simulink model "testexp1_cs"  (Simulink 8.8)
settings: Solver=ode5  StartTime=0.0  StopTime=inf  FixedStep=1/20  RelTol=1e-3
model workspace (MAT data in the model file):
  mbox_table.block_array(1).src = 'built-in/Subsystem'
  mbox_table.block_array(1).dest = 'testexp1_cs/Ford_FocusWagon_1'
  mbox_table.block_array(1).mode = 0
  mbox_table.block_array(2).src = 'simulink/Sinks/Out1'
  mbox_table.block_array(2).dest = 'testexp1_cs/Ford_FocusWagon_1/STATE_Ford_FocusWagon_1'
  mbox_table.block_array(2).mode = 0
  mbox_table.block_array(3).src = 'PreScanSimulinkLibrary/State'
  mbox_table.block_array(3).dest = 'testexp1_cs/STATE_Ford_FocusWagon_1'
  mbox_table.block_array(3).mode = 0
  mbox_table.block_array(4).src = 'PreScanSimulinkLibrary/SELF'
  mbox_table.block_array(4).dest = 'testexp1_cs/SELF_Ford_FocusWagon_1'
  mbox_table.block_array(4).mode = 0
  mbox_table.block_array(5).src = 'simulink/Sources/In1'
  mbox_table.block_array(5).dest = 'testexp1_cs/Ford_FocusWagon_1/SELF_Ford_FocusWagon_1'
  mbox_table.block_array(5).mode = 0
  mbox_table.block_array(6).src = 'PreScanSimulinkLibrary/DemuxSELF'
  mbox_table.block_array(6).dest = 'testexp1_cs/Ford_FocusWagon_1/SELF_Demux'
  mbox_table.block_array(6).mode = 0
  mbox_table.block_array(7).src = 'PreScanSimulinkLibrary/UserSpecified_Subsys'
  mbox_table.block_array(7).dest = 'testexp1_cs/Ford_FocusWagon_1/Dynamics_UserSpecified'
  mbox_table.block_array(7).mode = 0
  mbox_table.block_array(8).src = 'PreScanSimulinkLibrary/MuxState'
  mbox_table.block_array(8).dest = 'testexp1_cs/Ford_FocusWagon_1/Dynamics_UserSpecified/MuxState'
  mbox_table.block_array(8).mode = 0
  mbox_table.block_array(9).src = 'simulink/Sinks/Out1'
  mbox_table.block_array(9).dest = 'testexp1_cs/Ford_FocusWagon_1/Dynamics_UserSpecified/State'
  mbox_table.block_array(9).mode = 0
  mbox_table.block_array(10).src = 'built-in/Note'
  mbox_table.block_array(10).dest = 'testexp1_cs/Ford_FocusWagon_1/Dynamics_UserSpecified/For state mode ''Dynamic'' positions
    | are not taken into account, as they
    | are computed by integrating velocity.
    | Click annotation for Help.'
  mbox_table.block_array(10).mode = 0
  mbox_table.block_array(11).src = 'SimCoreLibrary/SimCoreConfiguration'
  mbox_table.block_array(11).dest = 'testexp1_cs/SimCoreConfiguration'
  mbox_table.block_array(11).mode = 0
  mbox_table.block_array(12).src = 'SimCoreLibrary/Actuators'
  mbox_table.block_array(12).dest = 'testexp1_cs/Actuators'
  mbox_table.block_array(12).mode = 0
  mbox_table.block_array(13).src = 'SimCoreLibrary/SetActuators'
  mbox_table.block_array(13).dest = 'testexp1_cs/SetActuators'
  mbox_table.block_array(13).mode = 0
  mbox_table.block_array(14).src = 'SimCoreLibrary/GetSensors'
  mbox_table.block_array(14).dest = 'testexp1_cs/GetSensors'
  mbox_table.block_array(14).mode = 0
  mbox_table.block_array(15).src = 'SimCoreLibrary/SimCoreInfo'
  mbox_table.block_array(15).dest = 'testexp1_cs/SimCoreInfo'
  mbox_table.block_array(15).mode = 0
  mbox_table.block_array(16).src = 'PreScanSimulinkLibrary/Regenerate'
  mbox_table.block_array(16).dest = 'testexp1_cs/Regenerate'
  mbox_table.block_array(16).mode = 0
  mbox_table.block_array(17).src = 'PreScanSimulinkLibrary/Record for Replay  '
  mbox_table.block_array(17).dest = 'testexp1_cs/Record for Replay  '
  mbox_table.block_array(17).mode = 0
  mbox_table.block_array(18).src = 'PreScanSimulinkLibrary/Open Useful Blocks'
  mbox_table.block_array(18).dest = 'testexp1_cs/Open Useful Blocks'
  mbox_table.block_array(18).mode = 0
  mbox_table.block_array(19).src = 'PreScanSimulinkLibrary/PreScan Options   '
  mbox_table.block_array(19).dest = 'testexp1_cs/PreScan Options   '
  mbox_table.block_array(19).mode = 0
  mbox_table.block_array(20).src = 'built-in/Note'
  mbox_table.block_array(20).dest = 'testexp1_cs/Version:                  '
  mbox_table.block_array(20).mode = 0
  mbox_table.block_array(21).src = 'built-in/Note'
  mbox_table.block_array(21).dest = 'testexp1_cs/7.5.1'
  mbox_table.block_array(21).mode = 0
  mbox_table.block_array(22).src = 'built-in/Note'
  mbox_table.block_array(22).dest = 'testexp1_cs/Author(s):                '
  mbox_table.block_array(22).mode = 0
  mbox_table.block_array(23).src = 'built-in/Note'
  mbox_table.block_array(23).dest = 'testexp1_cs/N.A.'
  mbox_table.block_array(23).mode = 0
  mbox_table.block_array(24).src = 'built-in/Note'
  mbox_table.block_array(24).dest = 'testexp1_cs/Descriptive text:      '
  mbox_table.block_array(24).mode = 0
  mbox_table.block_array(25).src = 'built-in/Note'
  mbox_table.block_array(25).dest = 'testexp1_cs/N.A.'
  mbox_table.block_array(25).mode = 0
  mbox_table.block_array(26).src = 'built-in/Note'
  mbox_table.block_array(26).dest = 'testexp1_cs/ID
    | 
    | 2'
  mbox_table.block_array(26).mode = 0
  mbox_table.block_array(27).src = 'built-in/Note'
  mbox_table.block_array(27).dest = 'testexp1_cs/OBU-Beacon ID
    | 
    | '
  mbox_table.block_array(27).mode = 0
  mbox_table.block_array(28).src = 'built-in/Note'
  mbox_table.block_array(28).dest = 'testexp1_cs/TypeID
    | 
    | 1'
  mbox_table.block_array(28).mode = 0
  mbox_table.block_array(29).src = 'built-in/Note'
  mbox_table.block_array(29).dest = 'testexp1_cs/TypeTag
    | 
    | Car'
  mbox_table.block_array(29).mode = 0
  mbox_table.block_array(30).src = 'built-in/Note'
  mbox_table.block_array(30).dest = 'testexp1_cs/SD
    | 
    | Y'
  mbox_table.block_array(30).mode = 0
  mbox_table.block_array(31).src = 'built-in/Note'
  mbox_table.block_array(31).dest = 'testexp1_cs/CD
    | 
    | N'
  mbox_table.block_array(31).mode = 0
  mbox_table.block_array(32).src = 'built-in/Note'
  mbox_table.block_array(32).dest = 'testexp1_cs/Name
    | 
    | Ford_FocusWagon_1'
  mbox_table.block_array(32).mode = 0
  mbox_table.block_array(33).src = 'built-in/Note'
  mbox_table.block_array(33).dest = 'testexp1_cs/Num ID       OBU-Beacon ID     Type ID      Type Tag             SD        CD             Name                          '
  mbox_table.block_array(33).mode = 0
  mbox_table.block_array(34).src = 'built-in/Ground'
  mbox_table.block_array(34).dest = 'testexp1_cs/Ford_FocusWagon_1/Ground_1'
  mbox_table.block_array(34).mode = 1
  mbox_table.block_array(35).src = 'built-in/Terminator'
  mbox_table.block_array(35).dest = 'testexp1_cs/Ford_FocusWagon_1/Terminator_1'
  mbox_table.block_array(35).mode = 1
  mbox_table.block_array(36).src = 'built-in/Ground'
  mbox_table.block_array(36).dest = 'testexp1_cs/Ford_FocusWagon_1/Dynamics_UserSpecified/Ground_1'
  mbox_table.block_array(36).mode = 1
  mbox_table.block_array(37).src = 'built-in/Ground'
  mbox_table.block_array(37).dest = 'testexp1_cs/Ford_FocusWagon_1/Dynamics_UserSpecified/Ground_2'
  mbox_table.block_array(37).mode = 1
  mbox_table.block_array(38).src = 'built-in/Ground'
  mbox_table.block_array(38).dest = 'testexp1_cs/Ford_FocusWagon_1/Dynamics_UserSpecified/Ground_3'
  mbox_table.block_array(38).mode = 1
  mbox_table.block_array(39).src = 'built-in/Ground'
  mbox_table.block_array(39).dest = 'testexp1_cs/Ford_FocusWagon_1/Dynamics_UserSpecified/Ground_4'
  mbox_table.block_array(39).mode = 1
  mbox_table.block_array(40).src = 'built-in/Ground'
  mbox_table.block_array(40).dest = 'testexp1_cs/Ford_FocusWagon_1/Dynamics_UserSpecified/Ground_5'
  mbox_table.block_array(40).mode = 1
  mbox_table.block_array(41).src = 'built-in/Ground'
  mbox_table.block_array(41).dest = 'testexp1_cs/Ford_FocusWagon_1/Dynamics_UserSpecified/Ground_6'
  mbox_table.block_array(41).mode = 1
  mbox_table.block_array(42).src = 'built-in/Ground'
  mbox_table.block_array(42).dest = 'testexp1_cs/Ford_FocusWagon_1/Dynamics_UserSpecified/Ground_7'
  mbox_table.block_array(42).mode = 1
  mbox_table.block_array(43).src = 'built-in/Ground'
  mbox_table.block_array(43).dest = 'testexp1_cs/Ford_FocusWagon_1/Dynamics_UserSpecified/Ground_8'
  mbox_table.block_array(43).mode = 1
  mbox_table.block_array(44).src = 'built-in/Ground'
  mbox_table.block_array(44).dest = 'testexp1_cs/Ford_FocusWagon_1/Dynamics_UserSpecified/Ground_9'
  mbox_table.block_array(44).mode = 1
  mbox_table.block_array(45).src = 'built-in/Terminator'
  mbox_table.block_array(45).dest = 'testexp1_cs/Ford_FocusWagon_1/Dynamics_UserSpecified/Terminator_1'
  mbox_table.block_array(45).mode = 1
  mbox_table.block_array(46).src = 'built-in/Terminator'
  mbox_table.block_array(46).dest = 'testexp1_cs/Ford_FocusWagon_1/Terminator_2'
  mbox_table.block_array(46).mode = 1
  mbox_table.block_array(47).src = 'built-in/Terminator'
  mbox_table.block_array(47).dest = 'testexp1_cs/Ford_FocusWagon_1/Terminator_3'
  mbox_table.block_array(47).mode = 1
  mbox_table.block_array(48).src = 'built-in/Terminator'
  mbox_table.block_array(48).dest = 'testexp1_cs/Ford_FocusWagon_1/Terminator_4'
  mbox_table.block_array(48).mode = 1
  mbox_table.block_array(49).src = 'built-in/Terminator'
  mbox_table.block_array(49).dest = 'testexp1_cs/Ford_FocusWagon_1/Terminator_5'
  mbox_table.block_array(49).mode = 1
  mbox_table.block_array(50).src = 'built-in/Terminator'
  mbox_table.block_array(50).dest = 'testexp1_cs/Ford_FocusWagon_1/Terminator_6'
  mbox_table.block_array(50).mode = 1
  mbox_table.block_array(51).src = 'built-in/Terminator'
  mbox_table.block_array(51).dest = 'testexp1_cs/Ford_FocusWagon_1/Terminator_7'
  mbox_table.block_array(51).mode = 1
  mbox_table.block_array(52).src = 'built-in/Terminator'
  mbox_table.block_array(52).dest = 'testexp1_cs/Ford_FocusWagon_1/Terminator_8'
  mbox_table.block_array(52).mode = 1
  mbox_table.block_array(53).src = 'built-in/Terminator'
  mbox_table.block_array(53).dest = 'testexp1_cs/Ford_FocusWagon_1/Terminator_9'
  mbox_table.block_array(53).mode = 1
  mbox_table.block_array(54).src = 'built-in/Terminator'
  mbox_table.block_array(54).dest = 'testexp1_cs/Ford_FocusWagon_1/Terminator_10'
  mbox_table.block_array(54).mode = 1
  mbox_table.block_array(55).src = 'built-in/Terminator'
  mbox_table.block_array(55).dest = 'testexp1_cs/Ford_FocusWagon_1/Terminator_11'
  mbox_table.block_array(55).mode = 1
  mbox_table.block_array(56).src = 'built-in/Terminator'
  mbox_table.block_array(56).dest = 'testexp1_cs/Ford_FocusWagon_1/Terminator_12'
  mbox_table.block_array(56).mode = 1
  mbox_table.block_array(57).src = 'built-in/Terminator'
  mbox_table.block_array(57).dest = 'testexp1_cs/Ford_FocusWagon_1/Terminator_13'
  mbox_table.block_array(57).mode = 1
  mbox_table.block_index : java.util.Hashtable (value not decoded)
  mbox_table.line_array(1).sys = 'testexp1_cs'
  mbox_table.line_array(1).line_id = 'L1'
  mbox_table.line_array(1).iport = 'STATE_Ford_FocusWagon_1/1'
  mbox_table.line_array(1).oport = 'Ford_FocusWagon_1/1'
  mbox_table.line_array(1).mode = 0
  mbox_table.line_array(2).sys = 'testexp1_cs'
  mbox_table.line_array(2).line_id = 'L2'
  mbox_table.line_array(2).iport = 'Ford_FocusWagon_1/1'
  mbox_table.line_array(2).oport = 'SELF_Ford_FocusWagon_1/1'
  mbox_table.line_array(2).mode = 0
  mbox_table.line_array(3).sys = 'testexp1_cs/Ford_FocusWagon_1'
  mbox_table.line_array(3).line_id = 'L3'
  mbox_table.line_array(3).iport = 'SELF_Demux/1'
  mbox_table.line_array(3).oport = 'SELF_Ford_FocusWagon_1/1'
  mbox_table.line_array(3).mode = 0
  mbox_table.line_array(4).sys = 'testexp1_cs/Ford_FocusWagon_1/Dynamics_UserSpecified'
  mbox_table.line_array(4).line_id = 'L4'
  mbox_table.line_array(4).iport = 'State/1'
  mbox_table.line_array(4).oport = 'MuxState/1'
  mbox_table.line_array(4).mode = 0
  mbox_table.line_array(5).sys = 'testexp1_cs/Ford_FocusWagon_1'
  mbox_table.line_array(5).line_id = 'L5'
  mbox_table.line_array(5).iport = 'STATE_Ford_FocusWagon_1/1'
  mbox_table.line_array(5).oport = 'Dynamics_UserSpecified/1'
  mbox_table.line_array(5).mode = 0
  mbox_table.line_array(6).sys = 'testexp1_cs/Ford_FocusWagon_1'
  mbox_table.line_array(6).line_id = 'l1'
  mbox_table.line_array(6).iport = 'Dynamics_UserSpecified/1'
  mbox_table.line_array(6).oport = 'Ground_1/1'
  mbox_table.line_array(6).mode = 1
  mbox_table.line_array(7).sys = 'testexp1_cs/Ford_FocusWagon_1'
  mbox_table.line_array(7).line_id = 'l2'
  mbox_table.line_array(7).iport = 'Terminator_1/1'
  mbox_table.line_array(7).oport = 'Dynamics_UserSpecified/2'
  mbox_table.line_array(7).mode = 1
  mbox_table.line_array(8).sys = 'testexp1_cs/Ford_FocusWagon_1/Dynamics_UserSpecified'
  mbox_table.line_array(8).line_id = 'l3'
  mbox_table.line_array(8).iport = 'MuxState/1'
  mbox_table.line_array(8).oport = 'Ground_1/1'
  mbox_table.line_array(8).mode = 1
  mbox_table.line_array(9).sys = 'testexp1_cs/Ford_FocusWagon_1/Dynamics_UserSpecified'
  mbox_table.line_array(9).line_id = 'l4'
  mbox_table.line_array(9).iport = 'MuxState/2'
  mbox_table.line_array(9).oport = 'Ground_2/1'
  mbox_table.line_array(9).mode = 1
  mbox_table.line_array(10).sys = 'testexp1_cs/Ford_FocusWagon_1/Dynamics_UserSpecified'
  mbox_table.line_array(10).line_id = 'l5'
  mbox_table.line_array(10).iport = 'MuxState/3'
  mbox_table.line_array(10).oport = 'Ground_3/1'
  mbox_table.line_array(10).mode = 1
  mbox_table.line_array(11).sys = 'testexp1_cs/Ford_FocusWagon_1/Dynamics_UserSpecified'
  mbox_table.line_array(11).line_id = 'l6'
  mbox_table.line_array(11).iport = 'MuxState/4'
  mbox_table.line_array(11).oport = 'Ground_4/1'
  mbox_table.line_array(11).mode = 1
  mbox_table.line_array(12).sys = 'testexp1_cs/Ford_FocusWagon_1/Dynamics_UserSpecified'
  mbox_table.line_array(12).line_id = 'l7'
  mbox_table.line_array(12).iport = 'MuxState/5'
  mbox_table.line_array(12).oport = 'Ground_5/1'
  mbox_table.line_array(12).mode = 1
  mbox_table.line_array(13).sys = 'testexp1_cs/Ford_FocusWagon_1/Dynamics_UserSpecified'
  mbox_table.line_array(13).line_id = 'l8'
  mbox_table.line_array(13).iport = 'MuxState/6'
  mbox_table.line_array(13).oport = 'Ground_6/1'
  mbox_table.line_array(13).mode = 1
  mbox_table.line_array(14).sys = 'testexp1_cs/Ford_FocusWagon_1/Dynamics_UserSpecified'
  mbox_table.line_array(14).line_id = 'l9'
  mbox_table.line_array(14).iport = 'MuxState/7'
  mbox_table.line_array(14).oport = 'Ground_7/1'
  mbox_table.line_array(14).mode = 1
  mbox_table.line_array(15).sys = 'testexp1_cs/Ford_FocusWagon_1/Dynamics_UserSpecified'
  mbox_table.line_array(15).line_id = 'l10'
  mbox_table.line_array(15).iport = 'MuxState/8'
  mbox_table.line_array(15).oport = 'Ground_8/1'
  mbox_table.line_array(15).mode = 1
  mbox_table.line_array(16).sys = 'testexp1_cs/Ford_FocusWagon_1/Dynamics_UserSpecified'
  mbox_table.line_array(16).line_id = 'l11'
  mbox_table.line_array(16).iport = 'MuxState/9'
  mbox_table.line_array(16).oport = 'Ground_9/1'
  mbox_table.line_array(16).mode = 1
  mbox_table.line_array(17).sys = 'testexp1_cs/Ford_FocusWagon_1/Dynamics_UserSpecified'
  mbox_table.line_array(17).line_id = 'l12'
  mbox_table.line_array(17).iport = 'Terminator_1/1'
  mbox_table.line_array(17).oport = 'Sine Wave/1'
  mbox_table.line_array(17).mode = 1
  mbox_table.line_array(18).sys = 'testexp1_cs/Ford_FocusWagon_1'
  mbox_table.line_array(18).line_id = 'l13'
  mbox_table.line_array(18).iport = 'Terminator_2/1'
  mbox_table.line_array(18).oport = 'SELF_Demux/1'
  mbox_table.line_array(18).mode = 1
  mbox_table.line_array(19).sys = 'testexp1_cs/Ford_FocusWagon_1'
  mbox_table.line_array(19).line_id = 'l14'
  mbox_table.line_array(19).iport = 'Terminator_3/1'
  mbox_table.line_array(19).oport = 'SELF_Demux/2'
  mbox_table.line_array(19).mode = 1
  mbox_table.line_array(20).sys = 'testexp1_cs/Ford_FocusWagon_1'
  mbox_table.line_array(20).line_id = 'l15'
  mbox_table.line_array(20).iport = 'Terminator_4/1'
  mbox_table.line_array(20).oport = 'SELF_Demux/3'
  mbox_table.line_array(20).mode = 1
  mbox_table.line_array(21).sys = 'testexp1_cs/Ford_FocusWagon_1'
  mbox_table.line_array(21).line_id = 'l16'
  mbox_table.line_array(21).iport = 'Terminator_5/1'
  mbox_table.line_array(21).oport = 'SELF_Demux/4'
  mbox_table.line_array(21).mode = 1
  mbox_table.line_array(22).sys = 'testexp1_cs/Ford_FocusWagon_1'
  mbox_table.line_array(22).line_id = 'l17'
  mbox_table.line_array(22).iport = 'Terminator_6/1'
  mbox_table.line_array(22).oport = 'SELF_Demux/5'
  mbox_table.line_array(22).mode = 1
  mbox_table.line_array(23).sys = 'testexp1_cs/Ford_FocusWagon_1'
  mbox_table.line_array(23).line_id = 'l18'
  mbox_table.line_array(23).iport = 'Terminator_7/1'
  mbox_table.line_array(23).oport = 'SELF_Demux/6'
  mbox_table.line_array(23).mode = 1
  mbox_table.line_array(24).sys = 'testexp1_cs/Ford_FocusWagon_1'
  mbox_table.line_array(24).line_id = 'l19'
  mbox_table.line_array(24).iport = 'Terminator_8/1'
  mbox_table.line_array(24).oport = 'SELF_Demux/7'
  mbox_table.line_array(24).mode = 1
  mbox_table.line_array(25).sys = 'testexp1_cs/Ford_FocusWagon_1'
  mbox_table.line_array(25).line_id = 'l20'
  mbox_table.line_array(25).iport = 'Terminator_9/1'
  mbox_table.line_array(25).oport = 'SELF_Demux/8'
  mbox_table.line_array(25).mode = 1
  mbox_table.line_array(26).sys = 'testexp1_cs/Ford_FocusWagon_1'
  mbox_table.line_array(26).line_id = 'l21'
  mbox_table.line_array(26).iport = 'Terminator_10/1'
  mbox_table.line_array(26).oport = 'SELF_Demux/9'
  mbox_table.line_array(26).mode = 1
  mbox_table.line_array(27).sys = 'testexp1_cs/Ford_FocusWagon_1'
  mbox_table.line_array(27).line_id = 'l22'
  mbox_table.line_array(27).iport = 'Terminator_11/1'
  mbox_table.line_array(27).oport = 'SELF_Demux/10'
  mbox_table.line_array(27).mode = 1
  mbox_table.line_array(28).sys = 'testexp1_cs/Ford_FocusWagon_1'
  mbox_table.line_array(28).line_id = 'l23'
  mbox_table.line_array(28).iport = 'Terminator_12/1'
  mbox_table.line_array(28).oport = 'SELF_Demux/11'
  mbox_table.line_array(28).mode = 1
  mbox_table.line_array(29).sys = 'testexp1_cs/Ford_FocusWagon_1'
  mbox_table.line_array(29).line_id = 'l24'
  mbox_table.line_array(29).iport = 'Terminator_13/1'
  mbox_table.line_array(29).oport = 'SELF_Demux/12'
  mbox_table.line_array(29).mode = 1
  mbox_table.line_index : java.util.Hashtable (value not decoded)
  mbox_table.next_linenr = 6
  mbox_table.next_termlinenr = 25
  model_closed = 0
  sim_status = 0
PreLoadFcn:
  | check_NUTS_defined;
  | 
  | assignin('base',['model_closed_' bdroot],false);
InitFcn:
  | PreScanExperimentInitFcn(bdroot)
StopFcn:
  | PreScanExperimentStopFcn(bdroot)
undefined symbols (not defined in the file): DiscIntNeverNeededParam, FromPrescan, IdealSensors, psi, vd, x, y
libraries: PreScanSimulinkLibrary x2, PreScanUsefulBlocks x1
CloseFcn:
  | evalin('base',['clear model_closed_' bdroot]);
settings Model: Creator=PRESCAN  LastModifiedBy=sgopalswamy
settings OptimizationCC: ExpressionDepthLimit=2147483647  InitFltsAndDblsToZero=on
settings DebuggingCC: SaveWithParameterizedLinksMsg=none  SignalResolutionControl=TryResolveAllWithWarning  MultiTaskDSMMsg=warning  MultiTaskCondExecSysMsg=none
settings GRTTargetCC: TargetFcnLib=ansi_tfl_tmw.mat

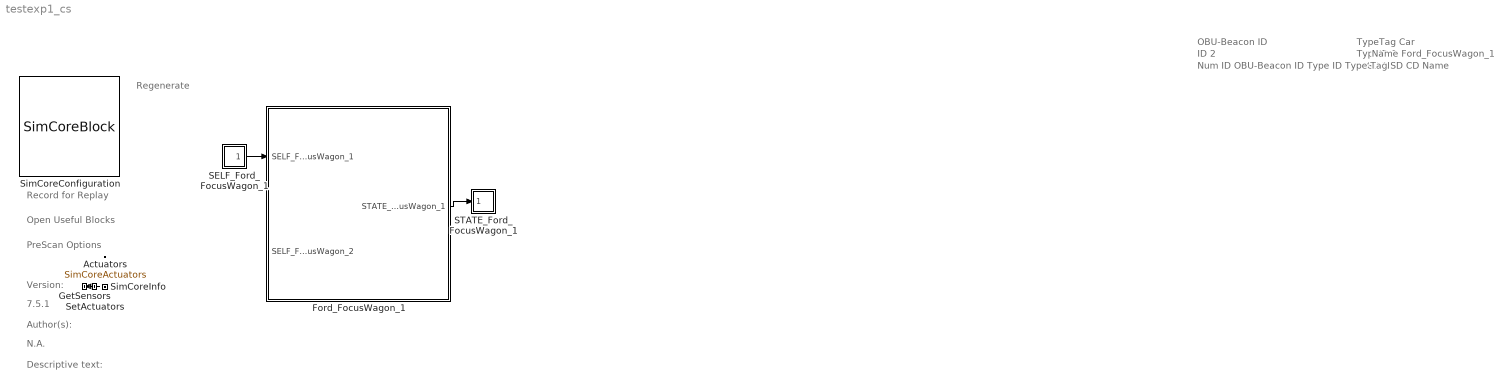
== system testexp1_cs ==
  note: Regenerate
  note: Record for Replay
  note: Open Useful Blocks
  note: PreScan Options
  note: Version:
  note: 7.5.1
  note: Author(s):
  note: N.A.
  note: Descriptive text:
  note: ID
      |
      | 2
  note: OBU-Beacon ID
  note: TypeID
      |
      | 1
  note: TypeTag
      |
      | Car
  note: SD
      |
      | Y
  note: CD
      |
      | N
  note: Name
      |
      | Ford_FocusWagon_1
  note: Num ID OBU-Beacon ID Type ID Type Tag SD CD Name
  Actuators : DataStoreMemory  DataStoreName=SimCoreActuators  InitialValue=zeros(15,1)  ShowAdditionalParam=off
  Ford_FocusWagon_1 : Subsystem  Tag=WorldObjectSubSystem  InitFcn=UniqueId = '14';
      mask Display: image(imread('Ford_FocusWagon.jpg'));color('white');text(0,0,' ID=2\n')
  GetSensors : Subsystem  Tag=GetSensors  Priority=2  mask(PreScan Simulation Core Block){NrOfSensors=8, TimeStep=1/20}
      mask prompts: NrOfSensors "Number of sensor values"; TimeStep "Timestep [s]"
      mask help:
      | Please do not remove this block from the PreScan compilation sheet,
      | as it contains essential configuration parameters for a PreScan simulation.
      settings: DeleteFcn=PreScanBlockDeleteFcn;
  SELF_Ford_FocusWagon_1 : Subsystem  Tag=SELF  Priority=3  mask(PreScan Source Block: SELF){PortName=SELF_Ford_FocusWagon_1, PortIndex=0, PortWidth=8, TimeStep=1/20}
      mask prompts: PortName "Auto-Assigned: Port Name [-]"; PortIndex "Auto-Assigned: Port Index [-]"; PortWidth "Auto-Assigned: Port Dimensions"; TimeStep "Auto-Assigned: Upload Period [s]"
      mask help:
      | The SELF port shows (state) information of the actor itself. The outputs are position in the experiment's axis system and the GPS coordinates, and the object's absolute velocity and compass heading.
      |
      | For more information, please click Help.
      settings: DeleteFcn=PreScanBlockDeleteFcn;
      mask Help: eval('openHelp(462)')
      mask Display: image(imread('GPS.png'))
  STATE_Ford_FocusWagon_1 : Subsystem  Tag=State  Priority=0  mask(PreScan Sink Block: State){x0=28.555984497070313, y0=57.32861328125, z0=0.5, Roll0=0, Pitch0=0, Yaw0=0, TimeStep=1/20}
      mask prompts: x0 "Ini x-position VEHICLE wrt GLOBAL axis system [m]"; y0 "Ini y-position VEHICLE wrt GLOBAL axis system [m]"; z0 "Ini z-position VEHICLE wrt GLOBAL axis system [m]"; Roll0 "Ini roll-angle BODY wrt VEHICLE axis system [deg]"; Pitch0 "Ini pitch-angle BODY wrt VEHICLE axis system [deg]"; Yaw0 "Ini yaw-angle VEHICLE wrt GLOBAL axis system [deg]"; TimeStep "Time Step [s]"
      mask help:
      | The Actor State contains a vector signal of size (9x1), containing the following signals:
      |
      | -  Position                  (x,y,z)                                     [m]
      | -  Velocity                  (vx,vy,vz)                               [m/s]
      | -  Angles                    (Roll, Pitch, Yaw)                   [rad]
      |
      | The Actor state is defined in the global axis system.
      | The state is superponed on the Initial position defined in the GUI.
      |
      | For more information, please click Help.
      settings: DeleteFcn=PreScanBlockDeleteFcn;
      mask Help: eval('openHelp(222)')
      mask Display: image(imread('State.png'))
  SetActuators : Subsystem  Tag=SetActuators  Priority=1  mask(PreScan Simulation Core Block){TimeStep=1/20, NrOfActuators=15}
      mask prompts: TimeStep "Timestep [s]"; NrOfActuators "Number of actuator values"
      mask help:
      | Please do not remove this block from the PreScan compilation sheet,
      | as it contains essential configuration parameters for a PreScan simulation.
      settings: DeleteFcn=PreScanBlockDeleteFcn;
  SimCoreConfiguration : M-S-Function  Tag=SimCoreConfiguration  Description=F795A25547817FA3818B88DB8D76BF7F6252BB85BC2E865D2A9867EEE6A99C6B  FunctionName=SimCoreBlock  Parameters=ExperimentXML PortsXML SimulationCore HostName CheckStart EnableLog RfR EnableGPUAccel ShowComputationTime  mask(PreScan Simulation Core Configurator){SimulationCore=NUTS, HostName=0, CheckStart=0, prescanversion='7.5.1', EnableLog=off, RfR=0, EnableGPUAccel=off, ShowComputationTime=off}
      mask prompts: SimulationCore "Simulation Core"; HostName "Simulation Host"; CheckStart "Show START Dialog"; prescanversion "PreScan Version"; EnableLog "Create TA Log"; RfR "Record for Replay"; EnableGPUAccel "Enable GPU Acceleration"; ShowComputationTime "Show ComputationTime Scope"
      mask help:
      | Please do not remove this block from the PreScan compilation sheet,
      | as it contains essential configuration parameter for a PreScan simulation.
      mask init:
      | model = bdroot;
      | ExperimentXML = [model(1:end-3) '.pex'];
      | PortsXML = [model '_ports.pcd'];
      settings: DeleteFcn=PreScanBlockDeleteFcn;  ModelCloseFcn=assignin('base',['model_closed_' bdroot],true);
      mask Help: eval('openHelp(812)')
      mask Display: image(imread('prescanlogo.ico'))
  SimCoreInfo : Subsystem  Tag=SimCoreInfo
  wires:
  SetActuators/1(dummy) -> GetSensors/1(dummy)
  Ford_FocusWagon_1/1(STATE_Ford_FocusWagon_1) -> STATE_Ford_FocusWagon_1/1(State)
  SELF_Ford_FocusWagon_1/1(U) -> Ford_FocusWagon_1/1(SELF_Ford_FocusWagon_1)

== system testexp1_cs/Ford_FocusWagon_1 ==
  SELF_Ford_FocusWagon_1 : Inport  Tag=SELFInport
  SELF_Ford_FocusWagon_2 : Inport  Tag=SELFInport  Port=2
  SingleVehicle_01 : Subsystem  mask{veh_struct=vd}
      mask prompts: veh_struct "Vehicle Parameter Structure"
      mask init:
      | set_param([gcb,'/Monitor/VehicleStateBusStorage'],'VariableName',[get_param(gcb,'MaskValueString'),'_DataVehicleBus']);
      | set_param([gcb,'/Monitor/ControllerMainBusStorage/ArbitratedActuationReqStorage'],'VariableName', ...
      |     [get_param(gcb,'MaskValueString'),'_DataControllerMain_ArbitrationActuationReq']);
      | set_param([gcb,'/Monitor/ControllerMainBusStorage/wpFollowerStorage'],'VariableName', ...
      |     [get_param(gcb,'MaskValueString'),'_DataControllerMain_wpFollower']);
      | set_param([gcb,'/Monitor/ControllerMainBusStorage/finalWayPointStorarge'],'VariableName', ...
      |     [get_param(gcb,'MaskValueString'),'_DataControllerMain_finalWayPoint']);
      | set_param([gcb,'/Monitor/ControllerMainBusStorage/currentWayPointStorage'],'VariableName', ...
      |     [get_param(gcb,'MaskValueString'),'_DataControllerMain_currentWayPoint']);
      | set_param([gcb,'/Monitor/ControllerMainBusStorage/wayPointArrayStorage'],'VariableName', ...
      |     [get_param(gcb,'MaskValueString'),'_DataControllerMain_wayPointArray']);
      | set_param([gcb,'/Monitor/ControllerMainBusStorage/selfAwareessBusStorage'],'VariableName', ...
      |     [get_param(gcb,'MaskValueString'),'_DataControllerMain_selfAwareessBus']);
      | set_param([gcb,'/Monitor/ControllerMainBusStorage/IdealSensorsStorage'],'VariableName', ...
      |     [get_param(gcb,'MaskValueString'),'_DataControllerMain_IdealSensors']);
      | set_param([gcb,'/Monitor/ControllerMainBusStorage/FromPrescanStorage'],'VariableName', ...
      |     [get_param(gcb,'MaskValueString'),'_DataControllerMain_FromPrescan']);
  STATE_Ford_FocusWagon_1 : Outport  Tag=StateOutport
  wires:
  SELF_Ford_FocusWagon_1/1 -> SingleVehicle_01/1(PrescanIn)
  SingleVehicle_01/1(VehicleStateBus) -> STATE_Ford_FocusWagon_1/1

== system testexp1_cs/GetSensors ==
  dummy : Inport
  GetSensors : M-S-Function  FunctionName=GetSensorsBlock  Parameters=TimeStep NrOfSensors
  tag scope: SimCoreSensors=global
  wires:
  GetSensors/1 -> [SimCoreSensors]
  dummy/1 -> GetSensors/1

== system testexp1_cs/SELF_Ford_FocusWagon_1 ==
  Selector : Selector  IndexMode=Zero-based  IndexOptions=Starting index (dialog)  Indices=PortIndex  OutputSizes=PortWidth(1)
  U : Outport
  wires:
  Selector/1 -> U/1
  [SimCoreSensors] -> Selector/1

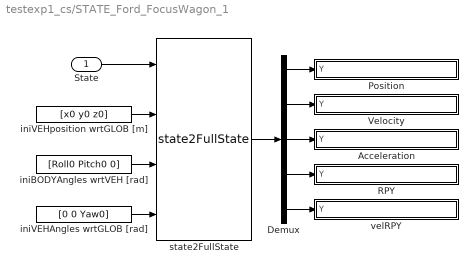
== system testexp1_cs/STATE_Ford_FocusWagon_1 ==
  State : Inport  SampleTime=TimeStep
  Acceleration : Subsystem  mask(ToSensorWorld){PortName=Acceleration_Ford_FocusWagon_1, PortIndex=6, PortWidth=3, TimeStep=1/20}
      mask prompts: PortName "Port Name [-]"; PortIndex "Index [-]"; PortWidth "Port Dimensions [-]"; TimeStep "Upload Period [s]"
      mask help: Sends signal(s) from Simulink to the Sensor World
      mask Help:
      | Sends signal(s) from Simulink to the Sensor World.
      | 
      | - Port Name [-]: specifies the name of the output terminal of the Simulink block.
      | - Index [-]: specifies the start position in the output vector sent to the Sensor World
      | - Port dimensions [-]: specifies the width (number of scalars) of the output port
      | - Upload period [s]: specifies the upload period (in seconds) of the port.
      mask Display: port_label('input', 1, PortName)
  Demux : Demux  Outputs=5
  Position : Subsystem  mask(ToSensorWorld){PortName=Position_Ford_FocusWagon_1, PortIndex=0, PortWidth=3, TimeStep=1/20}
      mask prompts: PortName "Port Name [-]"; PortIndex "Index [-]"; PortWidth "Port Dimensions [-]"; TimeStep "Upload Period [s]"
      mask help: Sends signal(s) from Simulink to the Sensor World
      mask Help:
      | Sends signal(s) from Simulink to the Sensor World.
      | 
      | - Port Name [-]: specifies the name of the output terminal of the Simulink block.
      | - Index [-]: specifies the start position in the output vector sent to the Sensor World
      | - Port dimensions [-]: specifies the width (number of scalars) of the output port
      | - Upload period [s]: specifies the upload period (in seconds) of the port.
      mask Display: port_label('input', 1, PortName)
  RPY : Subsystem  mask(ToSensorWorld){PortName=RPY_Ford_FocusWagon_1, PortIndex=9, PortWidth=3, TimeStep=1/20}
      mask prompts: PortName "Port Name [-]"; PortIndex "Index [-]"; PortWidth "Port Dimensions [-]"; TimeStep "Upload Period [s]"
      mask help: Sends signal(s) from Simulink to the Sensor World
      mask Help:
      | Sends signal(s) from Simulink to the Sensor World.
      | 
      | - Port Name [-]: specifies the name of the output terminal of the Simulink block.
      | - Index [-]: specifies the start position in the output vector sent to the Sensor World
      | - Port dimensions [-]: specifies the width (number of scalars) of the output port
      | - Upload period [s]: specifies the upload period (in seconds) of the port.
      mask Display: port_label('input', 1, PortName)
  Velocity : Subsystem  mask(ToSensorWorld){PortName=Velocity_Ford_FocusWagon_1, PortIndex=3, PortWidth=3, TimeStep=1/20}
      mask prompts: PortName "Port Name [-]"; PortIndex "Index [-]"; PortWidth "Port Dimensions [-]"; TimeStep "Upload Period [s]"
      mask help: Sends signal(s) from Simulink to the Sensor World
      mask Help:
      | Sends signal(s) from Simulink to the Sensor World.
      | 
      | - Port Name [-]: specifies the name of the output terminal of the Simulink block.
      | - Index [-]: specifies the start position in the output vector sent to the Sensor World
      | - Port dimensions [-]: specifies the width (number of scalars) of the output port
      | - Upload period [s]: specifies the upload period (in seconds) of the port.
      mask Display: port_label('input', 1, PortName)
  iniBODYAngles wrtVEH [rad] : Constant  Value=[Roll0 Pitch0 0]  SampleTime=TimeStep
  iniVEHAngles wrtGLOB [rad] : Constant  Value=[0 0 Yaw0]  SampleTime=TimeStep
  iniVEHposition wrtGLOB [m] : Constant  Value=[x0 y0 z0]  SampleTime=TimeStep
  state2FullState : PreScanSimulinkLibrary/state2FullState  SystemSampleTime=-1
  velRPY : Subsystem  mask(ToSensorWorld){PortName=velRPY_Ford_FocusWagon_1, PortIndex=12, PortWidth=3, TimeStep=1/20}
      mask prompts: PortName "Port Name [-]"; PortIndex "Index [-]"; PortWidth "Port Dimensions [-]"; TimeStep "Upload Period [s]"
      mask help: Sends signal(s) from Simulink to the Sensor World
      mask Help:
      | Sends signal(s) from Simulink to the Sensor World.
      | 
      | - Port Name [-]: specifies the name of the output terminal of the Simulink block.
      | - Index [-]: specifies the start position in the output vector sent to the Sensor World
      | - Port dimensions [-]: specifies the width (number of scalars) of the output port
      | - Upload period [s]: specifies the upload period (in seconds) of the port.
      mask Display: port_label('input', 1, PortName)
  wires:
  Demux/5 -> velRPY/1(Y)
  Demux/4 -> RPY/1(Y)
  Demux/3 -> Acceleration/1(Y)
  Demux/2 -> Velocity/1(Y)
  Demux/1 -> Position/1(Y)
  State/1 -> state2FullState/1
  state2FullState/1 -> Demux/1
  iniVEHposition wrtGLOB [m]/1 -> state2FullState/2
  iniBODYAngles wrtVEH [rad]/1 -> state2FullState/3
  iniVEHAngles wrtGLOB [rad]/1 -> state2FullState/4

== system testexp1_cs/SetActuators ==
  Bus Creator : BusCreator  Inputs=1
  Data Store Read : DataStoreRead  DataStoreName=SimCoreActuators  SampleTime=TimeStep
  SendActuators : M-S-Function  FunctionName=SendActuatorsBlock  Parameters=TimeStep NrOfActuators
  dummy : Outport
  tag scope: SimCoreInfo=global
  wires:
  Bus Creator/1 -> [SimCoreInfo]  "SimCore"
  SendActuators/2 -> Bus Creator/1  "ComputationTime[s]"
  SendActuators/1 -> dummy/1
  Data Store Read/1 -> SendActuators/1

== system testexp1_cs/SimCoreInfo ==
  Bus Selector : BusSelector  OutputSignals=ComputationTime[s]
  Time : Scope
  wires:
  Bus Selector/1 -> Time/1  "<ComputationTime[s]>"
  [SimCoreInfo] -> Bus Selector/1

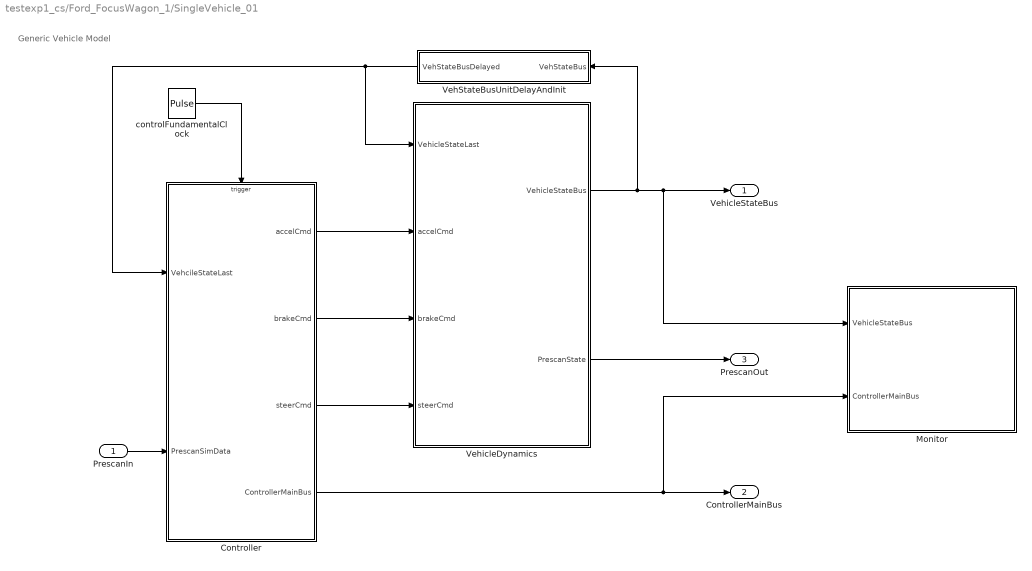
== system testexp1_cs/Ford_FocusWagon_1/SingleVehicle_01 ==
  note: Generic Vehicle Model
  PrescanIn : Inport
  Controller : Subsystem
  Monitor : Subsystem
  VehStateBusUnitDelayAndInit : Subsystem
  VehicleDynamics : Subsystem
  controlFundamentalClock : DiscretePulseGenerator  PulseType=Time based  Period=veh_struct.CONTROL_OS_SAMPLETIME  PulseWidth=5
  VehicleStateBus : Outport
  ControllerMainBus : Outport  Port=2
  PrescanOut : Outport  Port=3
  wires:
  PrescanIn/1 -> Controller/2(PrescanSimData)
  Controller/1(accelCmd) -> VehicleDynamics/2(accelCmd)
  Controller/2(brakeCmd) -> VehicleDynamics/3(brakeCmd)
  Controller/3(steerCmd) -> VehicleDynamics/4(steerCmd)
  Controller/4(ControllerMainBus) -> Monitor/2(ControllerMainBus), ControllerMainBus/1
  VehicleDynamics/2(PrescanState) -> PrescanOut/1
  VehicleDynamics/1(VehicleStateBus) -> VehStateBusUnitDelayAndInit/1(VehStateBus), VehicleStateBus/1, Monitor/1(VehicleStateBus)
  VehStateBusUnitDelayAndInit/1(VehStateBusDelayed) -> Controller/1(VehcileStateLast), VehicleDynamics/1(VehicleStateLast)
  controlFundamentalClock/1 -> Controller/Trigger

== system testexp1_cs/STATE_Ford_FocusWagon_1/Acceleration ==
  Y : Inport
  Assignment : Assignment  IndexMode=Zero-based  SampleTime=TimeStep  IndexOptions=Starting index (dialog)  Indices=PortIndex  OutputSizes=[1 1]
  Data Store Read : DataStoreRead  DataStoreName=SimCoreActuators  SampleTime=TimeStep
  Data Store Write : DataStoreWrite  DataStoreName=SimCoreActuators
  wires:
  Assignment/1 -> Data Store Write/1
  Data Store Read/1 -> Assignment/1
  Y/1 -> Assignment/2

== system testexp1_cs/STATE_Ford_FocusWagon_1/Position ==
  Y : Inport
  Assignment : Assignment  IndexMode=Zero-based  SampleTime=TimeStep  IndexOptions=Starting index (dialog)  Indices=PortIndex  OutputSizes=[1 1]
  Data Store Read : DataStoreRead  DataStoreName=SimCoreActuators  SampleTime=TimeStep
  Data Store Write : DataStoreWrite  DataStoreName=SimCoreActuators
  wires:
  Y/1 -> Assignment/2
  Data Store Read/1 -> Assignment/1
  Assignment/1 -> Data Store Write/1

== system testexp1_cs/STATE_Ford_FocusWagon_1/RPY ==
  Y : Inport
  Assignment : Assignment  IndexMode=Zero-based  SampleTime=TimeStep  IndexOptions=Starting index (dialog)  Indices=PortIndex  OutputSizes=[1 1]
  Data Store Read : DataStoreRead  DataStoreName=SimCoreActuators  SampleTime=TimeStep
  Data Store Write : DataStoreWrite  DataStoreName=SimCoreActuators
  wires:
  Assignment/1 -> Data Store Write/1
  Data Store Read/1 -> Assignment/1
  Y/1 -> Assignment/2

== system testexp1_cs/STATE_Ford_FocusWagon_1/Velocity ==
  Y : Inport
  Assignment : Assignment  IndexMode=Zero-based  SampleTime=TimeStep  IndexOptions=Starting index (dialog)  Indices=PortIndex  OutputSizes=[1 1]
  Data Store Read : DataStoreRead  DataStoreName=SimCoreActuators  SampleTime=TimeStep
  Data Store Write : DataStoreWrite  DataStoreName=SimCoreActuators
  wires:
  Assignment/1 -> Data Store Write/1
  Data Store Read/1 -> Assignment/1
  Y/1 -> Assignment/2

== system testexp1_cs/STATE_Ford_FocusWagon_1/velRPY ==
  Y : Inport
  Assignment : Assignment  IndexMode=Zero-based  SampleTime=TimeStep  IndexOptions=Starting index (dialog)  Indices=PortIndex  OutputSizes=[1 1]
  Data Store Read : DataStoreRead  DataStoreName=SimCoreActuators  SampleTime=TimeStep
  Data Store Write : DataStoreWrite  DataStoreName=SimCoreActuators
  wires:
  Assignment/1 -> Data Store Write/1
  Data Store Read/1 -> Assignment/1
  Y/1 -> Assignment/2

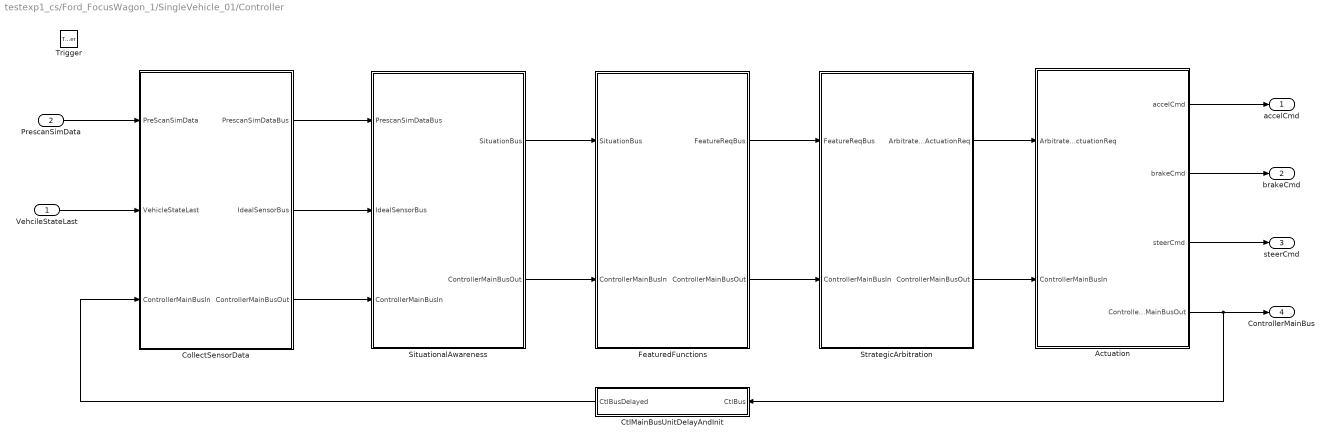
== system testexp1_cs/Ford_FocusWagon_1/SingleVehicle_01/Controller ==
  VehcileStateLast : Inport
  PrescanSimData : Inport  Port=2
  Trigger : TriggerPort  VariantControl=Variant  PortDimensions=1
  Actuation : Subsystem
  CollectSensorData : Subsystem
  CtlMainBusUnitDelayAndInit : Subsystem
  FeaturedFunctions : Subsystem
  SituationalAwareness : Subsystem
  StrategicArbitration : Subsystem
  accelCmd : Outport
  brakeCmd : Outport  Port=2
  steerCmd : Outport  Port=3
  ControllerMainBus : Outport  Port=4
  wires:
  PrescanSimData/1 -> CollectSensorData/1(PreScanSimData)
  Actuation/1(accelCmd) -> accelCmd/1
  Actuation/2(brakeCmd) -> brakeCmd/1
  Actuation/3(steerCmd) -> steerCmd/1
  StrategicArbitration/1(ArbitratedActuationReq) -> Actuation/1(ArbitratedActuationReq)
  StrategicArbitration/2(ControllerMainBusOut) -> Actuation/2(ControllerMainBusIn)
  FeaturedFunctions/2(ControllerMainBusOut) -> StrategicArbitration/2(ControllerMainBusIn)
  FeaturedFunctions/1(FeatureReqBus) -> StrategicArbitration/1(FeatureReqBus)
  SituationalAwareness/1(SituationBus) -> FeaturedFunctions/1(SituationBus)
  SituationalAwareness/2(ControllerMainBusOut) -> FeaturedFunctions/2(ControllerMainBusIn)
  CollectSensorData/3(ControllerMainBusOut) -> SituationalAwareness/3(ControllerMainBusIn)
  VehcileStateLast/1 -> CollectSensorData/2(VehicleStateLast)
  Actuation/4(ControllerMainBusOut) -> CtlMainBusUnitDelayAndInit/1(CtlBus), ControllerMainBus/1
  CtlMainBusUnitDelayAndInit/1(CtlBusDelayed) -> CollectSensorData/3(ControllerMainBusIn)
  CollectSensorData/1(PrescanSimDataBus) -> SituationalAwareness/1(PrescanSimDataBus)
  CollectSensorData/2(IdealSensorBus) -> SituationalAwareness/2(IdealSensorBus)

== system testexp1_cs/Ford_FocusWagon_1/SingleVehicle_01/Monitor ==
  VehicleStateBus : Inport
  ControllerMainBus : Inport  Port=2
  ControllerMainBusStorage : Subsystem
  VehicleStateBusStorage : ToWorkspace  VariableName=vd_DataVehicleBus  SaveFormat=Timeseries  SampleTime=-1
  wires:
  VehicleStateBus/1 -> VehicleStateBusStorage/1
  ControllerMainBus/1 -> ControllerMainBusStorage/1(ControllerMainBus)

== system testexp1_cs/Ford_FocusWagon_1/SingleVehicle_01/VehStateBusUnitDelayAndInit ==
  VehStateBus : Inport
  MATLAB Function : MATLAB Function  TreatAsAtomicUnit=on
  Memory : Memory  InheritSampleTime=on
  VehStateBusDelayed : Outport
  wires:
  Memory/1 -> MATLAB Function/1(u)
  VehStateBus/1 -> Memory/1
  MATLAB Function/1(y) -> VehStateBusDelayed/1

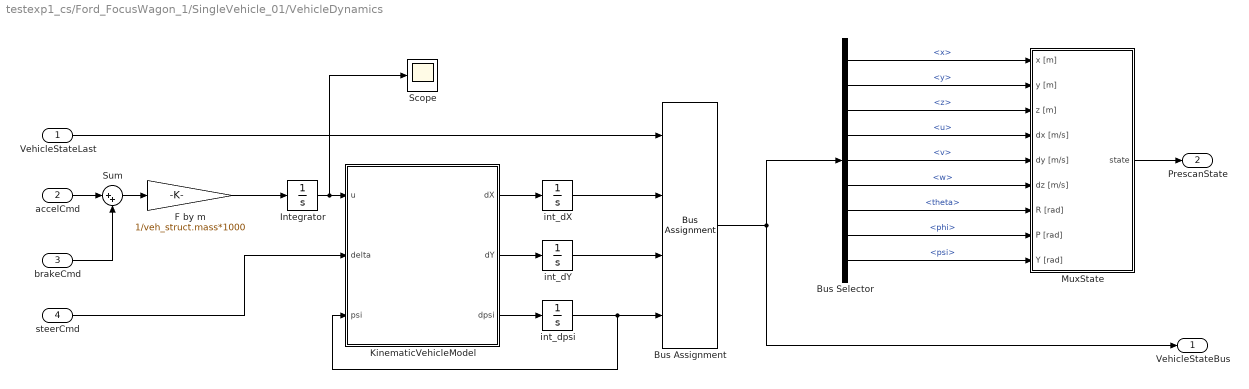
== system testexp1_cs/Ford_FocusWagon_1/SingleVehicle_01/VehicleDynamics ==
  VehicleStateLast : Inport
  accelCmd : Inport  Port=2
  brakeCmd : Inport  Port=3
  steerCmd : Inport  Port=4
  Bus Assignment : BusAssignment  AssignedSignals=x,y,psi
  Bus Selector : BusSelector  OutputSignals=x,y,z,u,v,w,theta,phi,psi
  F by m : Gain  Gain=1/veh_struct.mass*1000
  Integrator : Integrator  InitialCondition=veh_struct.init.u
  KinematicVehicleModel : MATLAB Function  TreatAsAtomicUnit=on
  MuxState : Subsystem  Tag=MuxState  mask(Empty Dynamics State Block){positioningmode=on, TimeStep=1/20}
      mask prompts: positioningmode "Positioning Mode"; TimeStep "Auto Assigned: Time Step [s]"
      mask help:
      | Build the state of an actor based on user input.
      | The user can either use positioning mode or dynamics mode.
      | - When using positioning mode the position and orientation of the actor are set directly based on the input. Expected input is relative to the initial position and orientation of the actor. It's also possible to specify the velocity of the actor, though this input isn't used, only passed on.
      | - When using dynamics mode the position input is ignored. Expected input is velocity and orientation. The velocity is relative the current orientation of the actor, while orientation is relative to its initial orientation. The position of the actor is calculated based on the velocity and orientation given.
      settings: DeleteFcn=PreScanBlockDeleteFcn;
  Scope : Scope
  Sum : Sum  Inputs=|++
  int_dX : Integrator  InitialCondition=veh_struct.init.X
  int_dY : Integrator  InitialCondition=veh_struct.init.Y
  int_dpsi : Integrator  InitialCondition=veh_struct.init.psi
  VehicleStateBus : Outport
  PrescanState : Outport  Port=2
  wires:
  MuxState/1(state) -> PrescanState/1
  Bus Assignment/1 -> Bus Selector/1, VehicleStateBus/1
  Bus Selector/3 -> MuxState/3(z [m])  "<z>"
  Bus Selector/4 -> MuxState/4(dx [m/s])  "<u>"
  Bus Selector/5 -> MuxState/5(dy [m/s])  "<v>"
  Bus Selector/6 -> MuxState/6(dz [m/s])  "<w>"
  Bus Selector/1 -> MuxState/1(x [m])  "<x>"
  Bus Selector/2 -> MuxState/2(y [m])  "<y>"
  Bus Selector/7 -> MuxState/7(R [rad])  "<theta>"
  Bus Selector/9 -> MuxState/9(Y [rad])  "<psi>"
  Bus Selector/8 -> MuxState/8(P [rad])  "<phi>"
  VehicleStateLast/1 -> Bus Assignment/1
  steerCmd/1 -> KinematicVehicleModel/2(delta)
  accelCmd/1 -> Sum/1
  brakeCmd/1 -> Sum/2
  Sum/1 -> F by m/1
  F by m/1 -> Integrator/1
  Integrator/1 -> Scope/1, KinematicVehicleModel/1(u)
  KinematicVehicleModel/2(dY) -> int_dY/1
  KinematicVehicleModel/1(dX) -> int_dX/1
  KinematicVehicleModel/3(dpsi) -> int_dpsi/1
  int_dX/1 -> Bus Assignment/2
  int_dY/1 -> Bus Assignment/3
  int_dpsi/1 -> Bus Assignment/4, KinematicVehicleModel/3(psi)

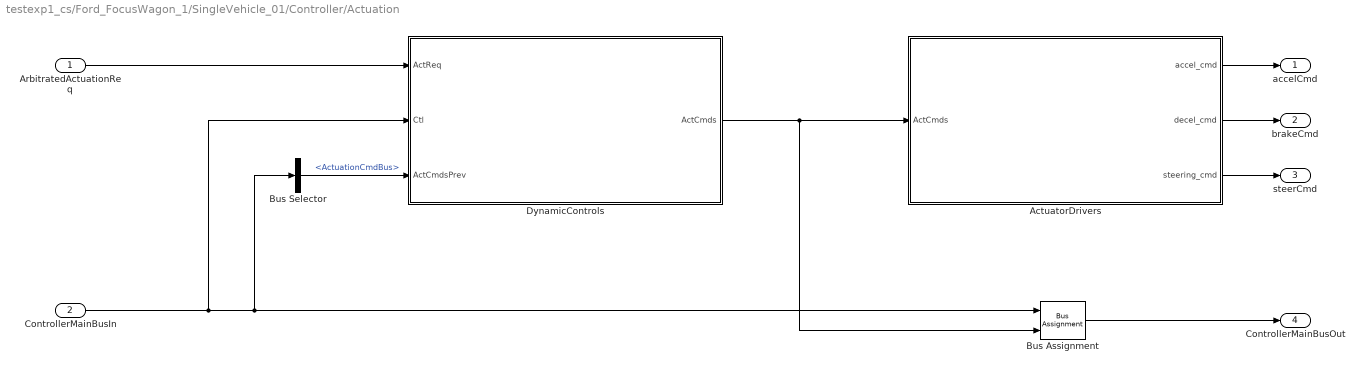
== system testexp1_cs/Ford_FocusWagon_1/SingleVehicle_01/Controller/Actuation ==
  ArbitratedActuationReq : Inport
  ControllerMainBusIn : Inport  Port=2
  ActuatorDrivers : MATLAB Function  TreatAsAtomicUnit=on
  Bus Assignment : BusAssignment  AssignedSignals=ActuationCmdBus
  Bus Selector : BusSelector  OutputSignals=ActuationCmdBus
  DynamicControls : MATLAB Function  TreatAsAtomicUnit=on
  accelCmd : Outport
  brakeCmd : Outport  Port=2
  steerCmd : Outport  Port=3
  ControllerMainBusOut : Outport  Port=4
  wires:
  ControllerMainBusIn/1 -> DynamicControls/2(Ctl), Bus Assignment/1, Bus Selector/1
  ArbitratedActuationReq/1 -> DynamicControls/1(ActReq)
  Bus Selector/1 -> DynamicControls/3(ActCmdsPrev)  "<ActuationCmdBus>"
  DynamicControls/1(ActCmds) -> ActuatorDrivers/1(ActCmds), Bus Assignment/2
  Bus Assignment/1 -> ControllerMainBusOut/1
  ActuatorDrivers/2(decel_cmd) -> brakeCmd/1
  ActuatorDrivers/1(accel_cmd) -> accelCmd/1
  ActuatorDrivers/3(steering_cmd) -> steerCmd/1

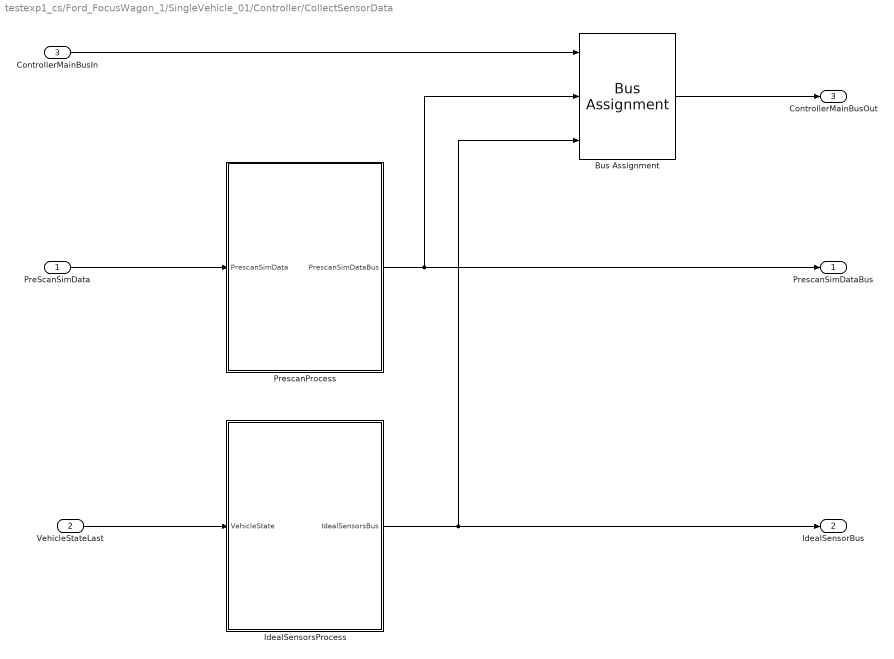
== system testexp1_cs/Ford_FocusWagon_1/SingleVehicle_01/Controller/CollectSensorData ==
  PreScanSimData : Inport
  VehicleStateLast : Inport  Port=2
  ControllerMainBusIn : Inport  Port=3
  Bus Assignment : BusAssignment  AssignedSignals=FromPrescan,IdealSensors
  IdealSensorsProcess : Subsystem
  PrescanProcess : Subsystem
  PrescanSimDataBus : Outport
  IdealSensorBus : Outport  Port=2
  ControllerMainBusOut : Outport  Port=3
  wires:
  PreScanSimData/1 -> PrescanProcess/1(PrescanSimData)
  PrescanProcess/1(PrescanSimDataBus) -> Bus Assignment/2, PrescanSimDataBus/1
  VehicleStateLast/1 -> IdealSensorsProcess/1(VehicleState)
  IdealSensorsProcess/1(IdealSensorsBus) -> IdealSensorBus/1, Bus Assignment/3
  Bus Assignment/1 -> ControllerMainBusOut/1
  ControllerMainBusIn/1 -> Bus Assignment/1

== system testexp1_cs/Ford_FocusWagon_1/SingleVehicle_01/Controller/CtlMainBusUnitDelayAndInit ==
  CtlBus : Inport
  MATLAB Function : MATLAB Function  TreatAsAtomicUnit=on
  Memory : Memory  InheritSampleTime=on
  CtlBusDelayed : Outport
  wires:
  Memory/1 -> MATLAB Function/1(u)
  CtlBus/1 -> Memory/1
  MATLAB Function/1(y) -> CtlBusDelayed/1

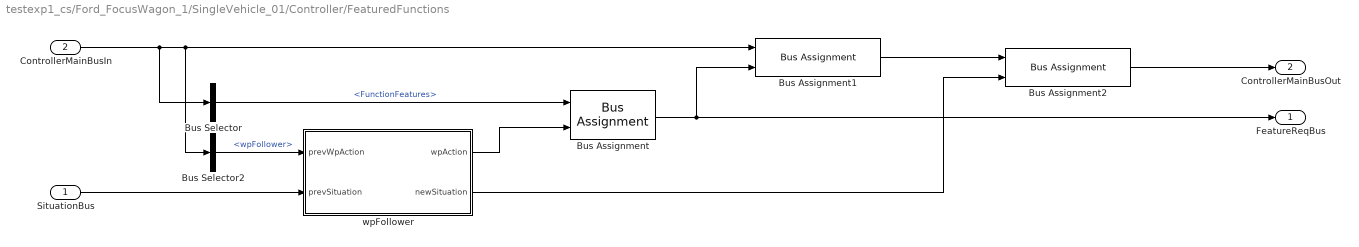
== system testexp1_cs/Ford_FocusWagon_1/SingleVehicle_01/Controller/FeaturedFunctions ==
  SituationBus : Inport
  ControllerMainBusIn : Inport  Port=2
  Bus Assignment : BusAssignment  AssignedSignals=wpFollower
  Bus Assignment1 : BusAssignment  AssignedSignals=FunctionFeatures
  Bus Assignment2 : BusAssignment  AssignedSignals=situationBus
  Bus Selector : BusSelector  OutputSignals=FunctionFeatures
  Bus Selector2 : BusSelector  OutputSignals=FunctionFeatures.wpFollower
  wpFollower : MATLAB Function  TreatAsAtomicUnit=on
  FeatureReqBus : Outport
  ControllerMainBusOut : Outport  Port=2
  wires:
  ControllerMainBusIn/1 -> Bus Selector/1, Bus Selector2/1, Bus Assignment1/1
  SituationBus/1 -> wpFollower/2(prevSituation)
  Bus Selector/1 -> Bus Assignment/1  "<FunctionFeatures>"
  wpFollower/1(wpAction) -> Bus Assignment/2
  Bus Assignment/1 -> Bus Assignment1/2, FeatureReqBus/1
  Bus Assignment1/1 -> Bus Assignment2/1
  wpFollower/2(newSituation) -> Bus Assignment2/2
  Bus Assignment2/1 -> ControllerMainBusOut/1
  Bus Selector2/1 -> wpFollower/1(prevWpAction)  "<wpFollower>"

== system testexp1_cs/Ford_FocusWagon_1/SingleVehicle_01/Controller/SituationalAwareness ==
  PrescanSimDataBus : Inport
  IdealSensorBus : Inport  Port=2
  ControllerMainBusIn : Inport  Port=3
  Bus Assignment : BusAssignment  AssignedSignals=situationBus
  Bus Selector : BusSelector  OutputSignals=situationBus
  situationAwareness : MATLAB Function  TreatAsAtomicUnit=on
  SituationBus : Outport
  ControllerMainBusOut : Outport  Port=2
  wires:
  ControllerMainBusIn/1 -> Bus Assignment/1, Bus Selector/1
  Bus Selector/1 -> situationAwareness/1(prevSituation)  "<situationBus>"
  PrescanSimDataBus/1 -> situationAwareness/2(prescanSimData)
  IdealSensorBus/1 -> situationAwareness/3(idealSensors)
  situationAwareness/1(newSituation) -> Bus Assignment/2, SituationBus/1
  Bus Assignment/1 -> ControllerMainBusOut/1

== system testexp1_cs/Ford_FocusWagon_1/SingleVehicle_01/Controller/StrategicArbitration ==
  FeatureReqBus : Inport
  ControllerMainBusIn : Inport  Port=2
  Arbitration : MATLAB Function  TreatAsAtomicUnit=on
  Bus Assignment : BusAssignment  AssignedSignals=ArbitratedActuationReq
  ArbitratedActuationReq : Outport
  ControllerMainBusOut : Outport  Port=2
  wires:
  ControllerMainBusIn/1 -> Bus Assignment/1
  FeatureReqBus/1 -> Arbitration/1(FunctionFeatures)
  Arbitration/1(ArbitratedReq) -> Bus Assignment/2, ArbitratedActuationReq/1
  Bus Assignment/1 -> ControllerMainBusOut/1

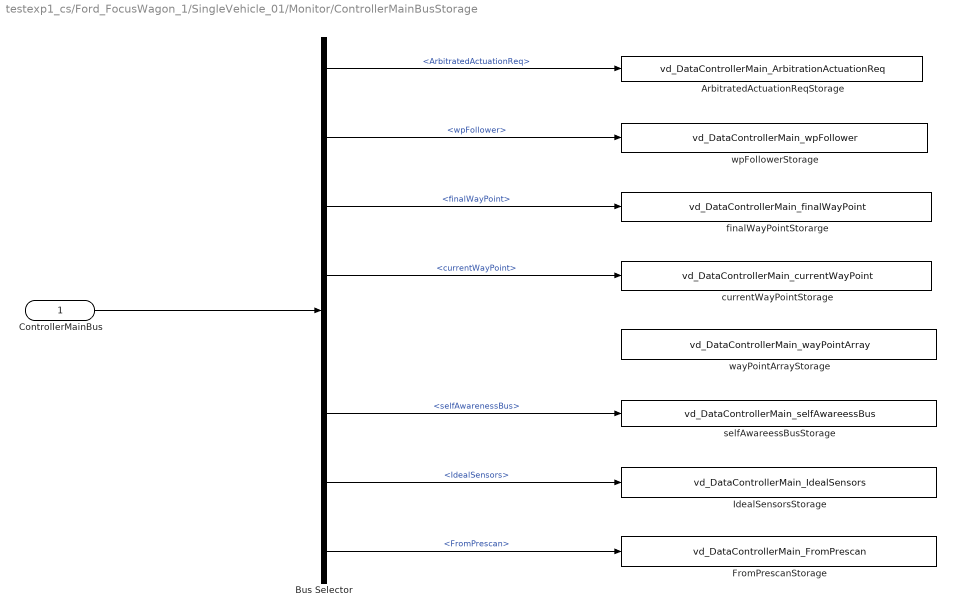
== system testexp1_cs/Ford_FocusWagon_1/SingleVehicle_01/Monitor/ControllerMainBusStorage ==
  ControllerMainBus : Inport
  ArbitratedActuationReqStorage : ToWorkspace  VariableName=vd_DataControllerMain_ArbitrationActuationReq  SaveFormat=Timeseries  SampleTime=-1
  Bus Selector : BusSelector  OutputSignals=ArbitratedActuationReq,FunctionFeatures.wpFollower,situationBus.wP.finalWayPoint,situationBus.wP.currentWayPoint,situationBus.wP.wayPointArray,situationBus.selfAwarenessBus,IdealSensors,FromPrescan
  FromPrescanStorage : ToWorkspace  VariableName=vd_DataControllerMain_FromPrescan  SaveFormat=Timeseries  SampleTime=-1
  IdealSensorsStorage : ToWorkspace  VariableName=vd_DataControllerMain_IdealSensors  SaveFormat=Timeseries  SampleTime=-1
  currentWayPointStorage : ToWorkspace  VariableName=vd_DataControllerMain_currentWayPoint  SaveFormat=Timeseries  SampleTime=-1
  finalWayPointStorarge : ToWorkspace  VariableName=vd_DataControllerMain_finalWayPoint  SaveFormat=Timeseries  SampleTime=-1
  selfAwareessBusStorage : ToWorkspace  VariableName=vd_DataControllerMain_selfAwareessBus  SaveFormat=Timeseries  SampleTime=-1
  wayPointArrayStorage : ToWorkspace  VariableName=vd_DataControllerMain_wayPointArray  SampleTime=-1
  wpFollowerStorage : ToWorkspace  VariableName=vd_DataControllerMain_wpFollower  SaveFormat=Timeseries  SampleTime=-1
  wires:
  ControllerMainBus/1 -> Bus Selector/1
  Bus Selector/1 -> ArbitratedActuationReqStorage/1  "<ArbitratedActuationReq>"
  Bus Selector/2 -> wpFollowerStorage/1  "<wpFollower>"
  Bus Selector/3 -> finalWayPointStorarge/1  "<finalWayPoint>"
  Bus Selector/8 -> FromPrescanStorage/1  "<FromPrescan>"
  Bus Selector/6 -> selfAwareessBusStorage/1  "<selfAwarenessBus>"
  Bus Selector/4 -> currentWayPointStorage/1  "<currentWayPoint>"
  Bus Selector/7 -> IdealSensorsStorage/1  "<IdealSensors>"

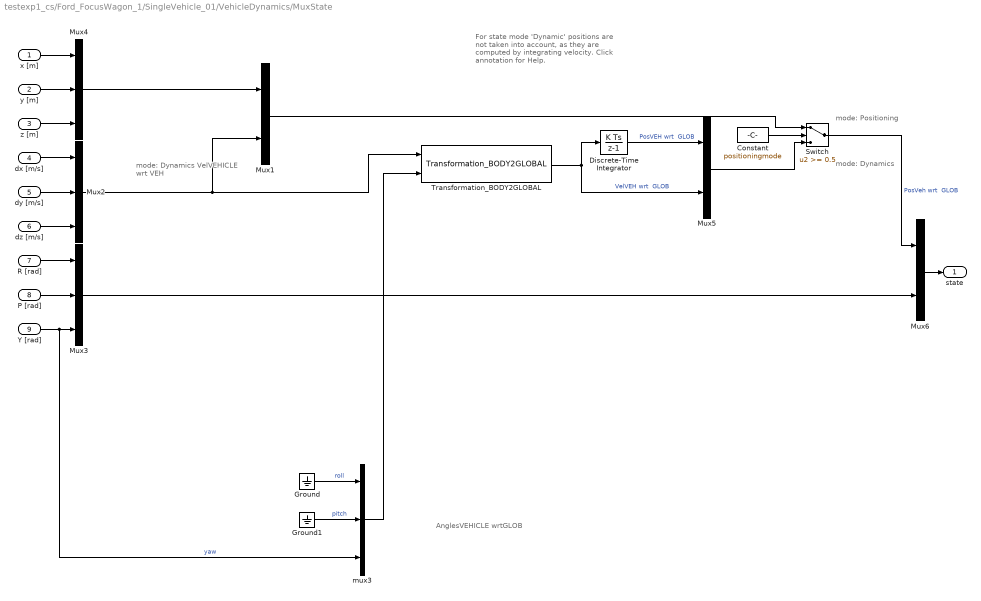
== system testexp1_cs/Ford_FocusWagon_1/SingleVehicle_01/VehicleDynamics/MuxState ==
  note: mode: Dynamics
  note: mode: Positioning
  note: mode: Dynamics
      | VelVEHICLE
      | wrt VEH
  note: AnglesVEHICLE
      | wrtGLOB
  note: For state mode 'Dynamic' positions
      | are not taken into account, as they
      | are computed by integrating velocity.
      | Click annotation for Help.
  x [m] : Inport  SampleTime=TimeStep
  y [m] : Inport  Port=2  SampleTime=TimeStep
  z [m] : Inport  Port=3  SampleTime=TimeStep
  dx [m/s] : Inport  Port=4  SampleTime=TimeStep
  dy [m/s] : Inport  Port=5  SampleTime=TimeStep
  dz [m/s] : Inport  Port=6  SampleTime=TimeStep
  R [rad] : Inport  Port=7  SampleTime=TimeStep
  P [rad] : Inport  Port=8  SampleTime=TimeStep
  Y [rad] : Inport  Port=9  SampleTime=TimeStep
  Constant : Constant  DisableCoverage=on  Value=positioningmode
  Discrete-Time Integrator : DiscreteIntegrator  SampleTime=TimeStep  ICPrevOutput=DiscIntNeverNeededParam  ICPrevScaledInput=DiscIntNeverNeededParam
  Ground : Ground
  Ground1 : Ground
  Mux1 : Mux  Inputs=[3 3]
  Mux2 : Mux  Inputs=3
  Mux3 : Mux  Inputs=3
  Mux4 : Mux  Inputs=3
  Mux5 : Mux  Inputs=[3 3]
  Mux6 : Mux  Inputs=[6 3]
  Switch : Switch  Threshold=0.5
  Transformation_BODY2GLOBAL : PreScanSimulinkLibrary/Simple_Vehicle_Dynamics/Chassis/MuxDynState/Transformation_BODY2GLOBAL
  mux3 : Mux  Inputs=3
  state : Outport
  wires:
  Constant/1 -> Switch/2
  Mux6/1 -> state/1
  Mux4/1 -> Mux1/1
  Mux5/1 -> Switch/3
  Mux1/1 -> Switch/1
  Switch/1 -> Mux6/1  "PosVeh wrt  GLOB"
  P [rad]/1 -> Mux3/2
  R [rad]/1 -> Mux3/1
  dz [m/s]/1 -> Mux2/3
  dy [m/s]/1 -> Mux2/2
  dx [m/s]/1 -> Mux2/1
  z [m]/1 -> Mux4/3
  y [m]/1 -> Mux4/2
  x [m]/1 -> Mux4/1
  Ground1/1 -> mux3/2  "pitch"
  Y [rad]/1 -> mux3/3, Mux3/3  "yaw"
  Mux3/1 -> Mux6/2
  Transformation_BODY2GLOBAL/1 -> Discrete-Time Integrator/1, Mux5/2  "VelVEH wrt  GLOB"
  mux3/1 -> Transformation_BODY2GLOBAL/2
  Ground/1 -> mux3/1  "roll"
  Mux2/1 -> Mux1/2, Transformation_BODY2GLOBAL/1
  Discrete-Time Integrator/1 -> Mux5/1  "PosVEH wrt  GLOB"

== system testexp1_cs/Ford_FocusWagon_1/SingleVehicle_01/Controller/CollectSensorData/IdealSensorsProcess ==
  VehicleState : Inport
  Bus Creator : BusCreator  Inputs=12  OutDataTypeStr=Bus: VehState
  Bus Selector : BusSelector  OutputSignals=x,y,z,theta,phi,psi,u,v,w,dtheta,dphi,dpsi
  IdealSensorsBus : Outport
  wires:
  VehicleState/1 -> Bus Selector/1
  Bus Selector/1 -> Bus Creator/1  "<x>"
  Bus Selector/8 -> Bus Creator/8  "<v>"
  Bus Selector/7 -> Bus Creator/7  "<u>"
  Bus Selector/10 -> Bus Creator/10  "<dtheta>"
  Bus Selector/11 -> Bus Creator/11  "<dphi>"
  Bus Selector/6 -> Bus Creator/6  "<psi>"
  Bus Selector/4 -> Bus Creator/4  "<theta>"
  Bus Selector/9 -> Bus Creator/9  "<w>"
  Bus Selector/2 -> Bus Creator/2  "<y>"
  Bus Selector/5 -> Bus Creator/5  "<phi>"
  Bus Selector/12 -> Bus Creator/12  "<dpsi>"
  Bus Selector/3 -> Bus Creator/3  "<z>"
  Bus Creator/1 -> IdealSensorsBus/1

== system testexp1_cs/Ford_FocusWagon_1/SingleVehicle_01/Controller/CollectSensorData/PrescanProcess ==
  PrescanSimData : Inport
  Bus Creator : BusCreator  Inputs=12  OutDataTypeStr=Bus: PrescanSimData
      settings: InheritFromInputs=off
  SELF_Demux : Subsystem  Tag=DemuxSELF  mask(PreScan Demux Block:){}
      settings: DeleteFcn=PreScanBlockDeleteFcn;
      mask Display:
      | port_label('output',1,'x [m]')
      | port_label('output',2,'y [m]')
      | port_label('output',3,'z [m]','texmode','on')
      | port_label('output',4,'Rotx [deg]','texmode','on')
      | port_label('output',5,'Roty [deg]','texmode','on')
      | port_label('output',6,'Rotz [deg]','texmode','on')
      | port_label('output',7,'GPS lat [deg]','texmode','on')
      | port_label('output',8,'GPS long [deg]','texmode','on')
      | port_label('output',9,'GPS alt [m]','texmode','on')
      | port_label('output',10,'Velocity [m/s]')
      | port_label('output',11,'Heading [deg]')
      | port_label('output',12,'Yaw rate [deg/s]')
  PrescanSimDataBus : Outport
  wires:
  SELF_Demux/1(x [m]) -> Bus Creator/1  "x"
  PrescanSimData/1 -> SELF_Demux/1(SELF)
  Bus Creator/1 -> PrescanSimDataBus/1
  SELF_Demux/2(y [m]) -> Bus Creator/2  "y"
  SELF_Demux/3(z [m]) -> Bus Creator/3  "z"
  SELF_Demux/4(rotx [deg]) -> Bus Creator/4  "Rotx"
  SELF_Demux/5(roty [deg]) -> Bus Creator/5  "Roty"
  SELF_Demux/9(GPS alt [m]) -> Bus Creator/9  "GPS_alt"
  SELF_Demux/8(GPS long [deg]) -> Bus Creator/8  "GPS_long"
  SELF_Demux/10(velocity [m/s]) -> Bus Creator/10  "u"
  SELF_Demux/6(rotz [deg]) -> Bus Creator/6  "Rotz"
  SELF_Demux/7(GPS lat [deg]) -> Bus Creator/7  "GPS_lat"
  SELF_Demux/11(heading [deg]) -> Bus Creator/11  "heading"
  SELF_Demux/12(yaw rate [deg/s]) -> Bus Creator/12  "Yaw_rate"

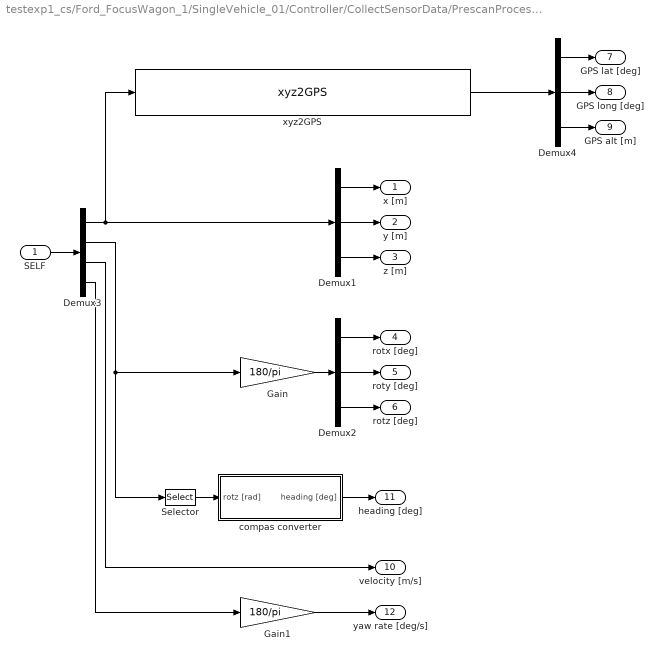
== system testexp1_cs/Ford_FocusWagon_1/SingleVehicle_01/Controller/CollectSensorData/PrescanProcess/SELF_Demux ==
  SELF : Inport
  Demux1 : Demux  Outputs=3
  Demux2 : Demux  Outputs=3
  Demux3 : Demux  Outputs=[3 3 1 1]
  Demux4 : Demux  Outputs=3
  Gain : Gain  Gain=180/pi
  Gain1 : Gain  Gain=180/pi
  Selector : Selector  InputPortWidth=3  IndexOptions=Index vector (dialog)  Indices=[3]  OutputSizes=1
  compas converter : Subsystem
  xyz2GPS : PreScanUsefulBlocks/xyz2GPS  CoordinateCount=1  GPS_base=[0.000000 0.000000 0.000]
  x [m] : Outport
  y [m] : Outport  Port=2
  z [m] : Outport  Port=3
  rotx [deg] : Outport  Port=4
  roty [deg] : Outport  Port=5
  rotz [deg] : Outport  Port=6
  GPS lat [deg] : Outport  Port=7
  GPS long [deg] : Outport  Port=8
  GPS alt [m] : Outport  Port=9
  velocity [m/s] : Outport  Port=10
  heading [deg] : Outport  Port=11
  yaw rate [deg/s] : Outport  Port=12
  wires:
  Demux3/4 -> Gain1/1
  Gain1/1 -> yaw rate [deg/s]/1
  Demux3/3 -> velocity [m/s]/1
  compas converter/1(heading [deg]) -> heading [deg]/1
  xyz2GPS/1 -> Demux4/1
  Demux4/3 -> GPS alt [m]/1
  Demux4/2 -> GPS long [deg]/1
  Demux4/1 -> GPS lat [deg]/1
  Demux3/2 -> Gain/1, Selector/1
  Demux3/1 -> xyz2GPS/1, Demux1/1
  SELF/1 -> Demux3/1
  Demux2/3 -> rotz [deg]/1
  Demux2/2 -> roty [deg]/1
  Demux2/1 -> rotx [deg]/1
  Demux1/3 -> z [m]/1
  Demux1/2 -> y [m]/1
  Demux1/1 -> x [m]/1
  Gain/1 -> Demux2/1
  Selector/1 -> compas converter/1(rotz [rad])

== system testexp1_cs/Ford_FocusWagon_1/SingleVehicle_01/Controller/CollectSensorData/PrescanProcess/SELF_Demux/compas converter ==
  rotz [rad] : Inport
  cart2compas : Subsystem
  rad2deg : Gain  Gain=180/pi
  heading [deg] : Outport
  wires:
  cart2compas/1(heading [deg]) -> heading [deg]/1
  rotz [rad]/1 -> rad2deg/1
  rad2deg/1 -> cart2compas/1(Angle [deg])

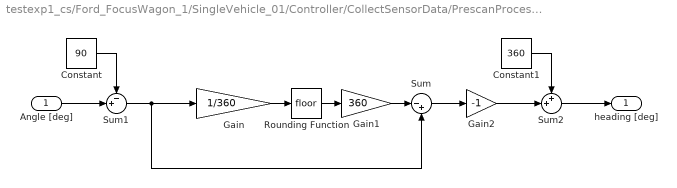
== system testexp1_cs/Ford_FocusWagon_1/SingleVehicle_01/Controller/CollectSensorData/PrescanProcess/SELF_Demux/compas converter/cart2compas ==
  Angle [deg] : Inport
  Constant : Constant  Value=90
  Constant1 : Constant  Value=360
  Gain : Gain  Gain=1/360
  Gain1 : Gain  Gain=360
  Gain2 : Gain  Gain=-1
  Rounding Function : Rounding
  Sum : Sum  Inputs=|-+
  Sum1 : Sum  Inputs=-+|
  Sum2 : Sum  Inputs=++|
  heading [deg] : Outport
  wires:
  Sum2/1 -> heading [deg]/1
  Constant1/1 -> Sum2/1
  Gain2/1 -> Sum2/2
  Constant/1 -> Sum1/1
  Sum1/1 -> Sum/2, Gain/1
  Sum/1 -> Gain2/1
  Angle [deg]/1 -> Sum1/2
  Gain1/1 -> Sum/1
  Rounding Function/1 -> Gain1/1
  Gain/1 -> Rounding Function/1

== matlab function Ford_FocusWagon_1/SingleVehicle_01/Controller/CtlMainBusUnitDelayAndInit/MATLAB Function ==
  data: u input double; y output Bus: ControllerMainBus; veh_struct parameter double
function y = DelayAndInitCtlBus(u, veh_struct)
coder.extrinsic('exist')
persistent a

y0 = struct;

y0.ActuationCmdBus = struct;
y0.ActuationCmdBus.steering_cmd = 0;
y0.ActuationCmdBus.decel_cmd = 0;
y0.ActuationCmdBus.accel_cmd = 0;

y0.ArbitratedActuationReq = struct;
y0.ArbitratedActuationReq.v_des = 0;
y0.ArbitratedActuationReq.a_des = 0;
y0.ArbitratedActuationReq.psi_des = 0;
y0.ArbitratedActuationReq.dpsi_des = 0;


y0.FunctionFeatures = struct;
y0.FunctionFeatures.wpFollower = struct;
y0.FunctionFeatures.wpFollower.v_des = 0;
y0.FunctionFeatures.wpFollower.a_des = 0;
y0.FunctionFeatures.wpFollower.psi_des = 0;
y0.FunctionFeatures.wpFollower.dpsi_des = 0;


y0.situationBus = struct;
y0.situationBus.wP = struct;

y0.situationBus.wP.finalWayPoint = struct;
y0.situationBus.wP.finalWayPoint.x = 0;
y0.situationBus.wP.finalWayPoint.y = 0;
y0.situationBus.wP.finalWayPoint.z = 0;
y0.situationBus.wP.finalWayPoint.treach = 0;

y0.situationBus.wP.currentWayPoint = struct;
y0.situationBus.wP.currentWayPoint.x = 0;
y0.situationBus.wP.currentWayPoint.y = 0;
y0.situationBus.wP.currentWayPoint.z = 0;
y0.situationBus.wP.currentWayPoint.treach = 0;

y0.situationBus.wP.finalWayPointIndex = uint16(1);
y0.situationBus.wP.currentWayPointIndex = uint16(10);

%y0.situationBus.wP.wayPointArray = struct;
wPArray = struct;
wPArray.x = 0;
wPArray.y = 0;
wPArray.z = 0;
wPArray.treach = 0;
y0.situationBus.wP.wayPointArray = repmat(wPArray,100,1);


y0.situationBus.selfAwarenessBus = struct;
y0.situationBus.selfAwarenessBus.x = 0;
y0.situationBus.selfAwarenessBus.y = 0;
y0.situationBus.selfAwarenessBus.z = 0;
y0.situationBus.selfAwarenessBus.theta = 0;
y0.situationBus.selfAwarenessBus.phi = 0;
y0.situationBus.selfAwarenessBus.psi = 0;
y0.situationBus.selfAwarenessBus.u = 0;
y0.situationBus.selfAwarenessBus.v = 0;
y0.situationBus.selfAwarenessBus.w = 0;
y0.situationBus.selfAwarenessBus.dtheta = 0;
y0.situationBus.selfAwarenessBus.dphi = 0;
y0.situationBus.selfAwarenessBus.dpsi = 0;
y0.IdealSensors = struct;
y0.IdealSensors.x = 0;
y0.IdealSensors.y = 0;
y0.IdealSensors.z = 0;
y0.IdealSensors.theta = 0;
y0.IdealSensors.phi = 0;
y0.IdealSensors.psi = 0;
y0.IdealSensors.u = 0;
y0.IdealSensors.v = 0;
y0.IdealSensors.w = 0;
y0.IdealSensors.dtheta = 0;
y0.IdealSensors.dphi = 0;
y0.IdealSensors.dpsi = 0;
y0.FromPrescan = struct;
y0.FromPrescan.x = 0;
y0.FromPrescan.y = 0;
y0.FromPrescan.z = 0;
y0.FromPrescan.Rotx = 0;
y0.FromPrescan.Roty = 0;
y0.FromPrescan.Rotz = 0;
y0.FromPrescan.GPS_lat = 0;
y0.FromPrescan.GPS_long = 0;
y0.FromPrescan.u = 0;
y0.FromPrescan.GPS_alt = 0;
y0.FromPrescan.heading = 0;
y0.FromPrescan.Yaw_rate = 0;



if isempty(a)
    a = 1;
    y = y0;
    y.situationBus.wP.wayPointArray = veh_struct.initialWayPointsArray;
    y.situationBus.wP.currentWayPointIndex = veh_struct.initialCurrentWayPointIndex;
    y.situationBus.wP.finalWayPointIndex = veh_struct.initialFinalWayPointIndex;

else
    y = u;
end

== matlab function Ford_FocusWagon_1/SingleVehicle_01/VehStateBusUnitDelayAndInit/MATLAB Function ==
  data: u input double; y output Bus: VehState
function y = DelayAndInitVehState(u)
persistent a
y0 = struct;
y0.x = 1;
y0.y = 2;
y0.z = 0;
y0.theta = 0;
y0.phi = 0;
y0.psi = 0;
y0.u = 0;
y0.v = 0;
y0.w = 0;
y0.dtheta = 0;
y0.dphi = 0;
y0.dpsi = 0;

%y0 = VehState_MATLABStruct;
if isempty(a)
    a = 1;
    y = y0;
else
    y = u;
end

== matlab function Ford_FocusWagon_1/SingleVehicle_01/Controller/SituationalAwareness/situationAwareness ==
  data: prevSituation input Bus: situationBus; newSituation output Bus: situationBus; prescanSimData input Bus: PrescanSimData; idealSensors input Bus: VehState; veh_struct parameter double
function newSituation = calcSituationAwareness(prevSituation,prescanSimData,idealSensors, veh_struct)

newSituation = prevSituation;


newSituation.selfAwarenessBus.x = idealSensors.x;
newSituation.selfAwarenessBus.y = idealSensors.y;
newSituation.selfAwarenessBus.z = idealSensors.z;
newSituation.selfAwarenessBus.theta = idealSensors.theta;
newSituation.selfAwarenessBus.phi = idealSensors.phi;
newSituation.selfAwarenessBus.psi = idealSensors.psi;
newSituation.selfAwarenessBus.u = idealSensors.u;
newSituation.selfAwarenessBus.v = idealSensors.v;
newSituation.selfAwarenessBus.w = idealSensors.w;
newSituation.selfAwarenessBus.dtheta = idealSensors.dtheta;
newSituation.selfAwarenessBus.dphi = idealSensors.dphi;
newSituation.selfAwarenessBus.dpsi = idealSensors.dpsi;


end

== matlab function Ford_FocusWagon_1/SingleVehicle_01/Controller/FeaturedFunctions/wpFollower ==
  data: prevWpAction input Bus: wpFollower; prevSituation input Bus: situationBus; wpAction output Bus: wpFollower; veh_struct parameter double; newSituation output Bus: situationBus
function [wpAction, newSituation] = wpFollower(prevWpAction, prevSituation, veh_struct)

currentIndex = prevSituation.wP.currentWayPointIndex;
if currentIndex < 1
    currentIndex = uint16(1);
end
finalIndex = prevSituation.wP.finalWayPointIndex;

xd = prevSituation.wP.wayPointArray(currentIndex).x;
yd = prevSituation.wP.wayPointArray(currentIndex).y;
xa = prevSituation.selfAwarenessBus.x;
ya = prevSituation.selfAwarenessBus.y;
howClose = norm([xd-xa, yd-ya]);

if howClose < veh_struct.wpControl.wayPointThreshold
    if (currentIndex == finalIndex)
        currentIndex = uint16(1);
    else
        currentIndex = uint16(currentIndex + 1);
    end
end

newSituation = prevSituation;
newSituation.wP.currentWayPointIndex = uint16(currentIndex);
newSituation.wP.currentWayPoint.x = newSituation.wP.wayPointArray(currentIndex).x;
newSituation.wP.currentWayPoint.y = newSituation.wP.wayPointArray(currentIndex).y;
newSituation.wP.currentWayPoint.z = newSituation.wP.wayPointArray(currentIndex).z;
newSituation.wP.currentWayPoint.treach = newSituation.wP.wayPointArray(currentIndex).treach;

v_des_raw = min(veh_struct.wpControl.v_des_max, howClose / veh_struct.wpControl.howClose_saturate * veh_struct.wpControl.v_des_max);
psi_des_raw = atan2((yd-ya),(xd-xa));

% if psi_des_raw < 0
%     
%     dbg = 1;
%     
% end
    

v_des_old = prevWpAction.v_des;
psi_des_old = prevWpAction.psi_des;

a_des = veh_struct.wpControl.v_des_filter.lambda * (v_des_raw - v_des_old);
v_des = v_des_old + veh_struct.CONTROL_OS_SAMPLETIME * a_des;

dpsi_des = veh_struct.wpControl.psi_des_filter.lambda * (psi_des_raw - psi_des_old);
psi_des = psi_des_old + veh_struct.CONTROL_OS_SAMPLETIME * dpsi_des;
% psi_des = mod(psi_des, 2 * pi);


wpAction.v_des = v_des;
wpAction.a_des = a_des;
wpAction.psi_des = psi_des;
wpAction.dpsi_des = dpsi_des;

end

== matlab function Ford_FocusWagon_1/SingleVehicle_01/Controller/StrategicArbitration/Arbitration ==
  data: FunctionFeatures input Bus: FunctionFeatures; ArbitratedReq output Bus: ArbitratedActuationReq
function ArbitratedReq = Arbitrate(FunctionFeatures)

ArbitratedReq.v_des = FunctionFeatures.wpFollower.v_des;
ArbitratedReq.a_des = FunctionFeatures.wpFollower.a_des;
ArbitratedReq.psi_des = FunctionFeatures.wpFollower.psi_des;
ArbitratedReq.dpsi_des = FunctionFeatures.wpFollower.dpsi_des;

end

== matlab function Ford_FocusWagon_1/SingleVehicle_01/Controller/Actuation/DynamicControls ==
  data: ActReq input Bus: ArbitratedActuationReq; Ctl input Bus: ControllerMainBus; ActCmds output Bus: ActuationCmdBus; ActCmdsPrev input Bus: ActuationCmdBus
function ActCmds  = fcn(ActReq, Ctl, ActCmdsPrev)

v_des = ActReq.v_des;
a_des = ActReq.a_des;
psi_des = ActReq.psi_des;
dpsi_des = ActReq.dpsi_des;

% ActCmds = ActCmdsPrev;
% ActCmds.accel_cmd = 0;
% ActCmds.decel_cmd = 0;
% ActCmds.steering_cmd = 0.1;

ActCmds = ActCmdsPrev;

if a_des >= 0
    ActCmds.accel_cmd = ActReq.a_des;
    ActCmds.decel_cmd = 0;
else
    ActCmds.accel_cmd = 0;
    ActCmds.decel_cmd = ActReq.a_des;
end

psi_des = unwrap(psi_des);
Ctl.IdealSensors.psi = unwrap(Ctl.IdealSensors.psi);

ActCmds.steering_cmd = 3.5*(psi_des - Ctl.IdealSensors.psi);

== matlab function Ford_FocusWagon_1/SingleVehicle_01/VehicleDynamics/KinematicVehicleModel ==
  data: u input double; delta input double; dX output double; psi input double; dY output double; dpsi output double; veh_struct parameter double
function [dX,dY,dpsi] = fcn(u,delta, psi, veh_struct)

lf = veh_struct.lf;
lr = veh_struct.lr;

% psi = unwrap(psi);
% delta = unwrap(delta);

beta = atan( lr /(lf + lr) * tan(delta));

% beta = unwrap(beta);

dX = u * cos(psi + beta);
dY = u * sin(psi + beta);
dpsi = u / lr * sin(beta);

== matlab function Ford_FocusWagon_1/SingleVehicle_01/Controller/Actuation/ActuatorDrivers ==
  data: ActCmds input Bus: ActuationCmdBus; accel_cmd output double; decel_cmd output double; steering_cmd output double
function [accel_cmd, decel_cmd, steering_cmd]  = fcn(ActCmds)

accel_cmd = ActCmds.accel_cmd;
decel_cmd = ActCmds.decel_cmd;
steering_cmd = ActCmds.steering_cmd;

end
